simulink model " PV_PEM_indirect"  (R2026a)
settings: Solver=ode15s  StopTime=sim_t  MaxStep=1e-5
values from neighbouring files (symbols this model uses):
  Ra_stack = Ra   * N    (= 0.02301)    [ PV_PEM_indirect.m]    (also in PV_PEM_indirect.m = 0.02832)
  Rc_stack = Rc   * N    (= 0.0065)    [ PV_PEM_indirect.m]    (also in PV_PEM_indirect.m = 0.008)
  Rint_stack = Rint * N    (= 0.112749)    [ PV_PEM_indirect.m]    (also in PV_PEM_indirect.m = 0.138768)
  sample_output_time = 1e-2    (= 0.01)    [ PV_PEM_indirect.m]    (also in PV_PEM_indirect.m = Irr_stair_tsamp)
  Ts = Irr_stair_tsamp / N_sw_per_step    [PV_PEM_indirect.m]
  Tsc = 1e-5    (= 1e-05)    [ PV_PEM_indirect.m]    (also in PV_PEM_indirect.m = 5e-05)
libraries: fl_lib x16, nesl_utility x15, ee_lib x3, simulink x2, eeDcDcVoltageController x1, eePwmGenerator x1
settings Model: SimulationMode=accelerator  Creator=hanna  LastModifiedBy=Diamantis
settings SimscapeCC: SimscapeNominalValues="[{\"value\":\"1\",\"unit\":\"A\"},{\"value\":\"1\",\"unit\":\"bar\"},{\"value\":\"1\",\"unit\":\"cm^2\"},{\"value\":\"1\",\"unit\":\"cm^3/s\"},{\"value\":\"1\",\"unit\":\"kJ/kg\"},{\"value\":\"1\",\"unit\":\"kW\"},{\"value\":\"1\",\"unit\":\"l\"},{\"value\":\"1\",\"unit\":\"N\"},{\"value\":\"1\",\"unit\":\"N*m\"},{\"value\":\"1\",\"unit\":\"V\"}]"  SimscapeLogType=none  SimscapeLogDataHistory=5000.0

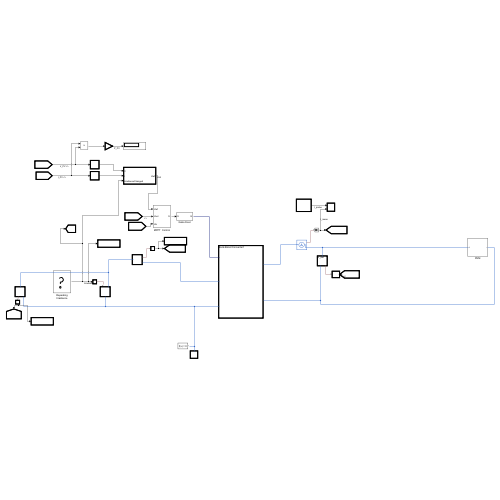
[thumbnail: Simulink's stored preview of the top-level diagram]
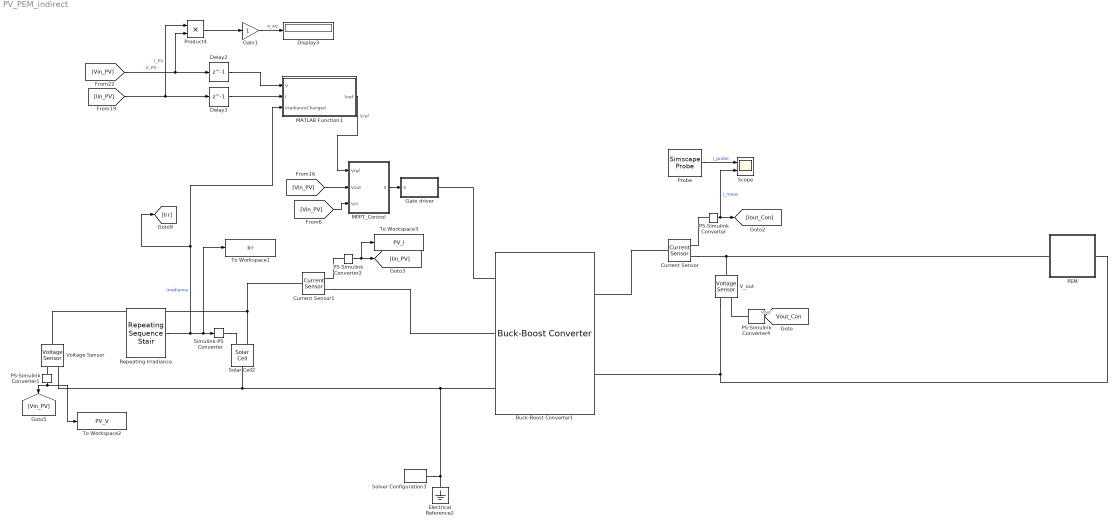
== system  PV_PEM_indirect ==
  Buck-Boost Converter1 : ee_lib/Semiconductors & Converters/Converters/Buck-Boost Converter  port_option=ee.enum.controlport.ps  device_type=4  Vf=0.8 V  Ron=0.001 Ohm  Rds=Ron Ohm  Goff=Conductance 1/Ohm  Vgt=1 V  Vgt_off=-1 V  Ih=1 A  Vth=Vth V  K=0  diode_param=2  diode_Vf=Vforward V  diode_Ron=1e-9 Ohm  diode_Goff=1e-6 1/Ohm  diode_C=50 nF  diode_iRM=5 A  diode_iF=300 A  diode_idot=-50 A/us  diode_trr_param=1  diode_trr_factor=3  diode_trr=0.5 us  diode_Qrr=1500 s*uA  Lf=L_conv H  Rl=0 Ohm  Cf=C_conv F  Rf=0 Ohm  snubber_type=1  Cs=1e-7 F  Rs=0.1 Ohm  iL_specify=off  iL_priority=High  iL=0 A  iL_nominal_specify=off  iL_nominal_value=1  iL_nominal_unit=A  vc_specify=off  vc_priority=High  vc=0 V  vc_nominal_specify=off  vc_nominal_value=1  vc_nominal_unit=V
  Current Sensor : fl_lib/Electrical/Electrical Sensors/Current Sensor
  Current Sensor1 : fl_lib/Electrical/Electrical Sensors/Current Sensor
  Delay2 : Delay  DelayLength=1
  Delay3 : Delay  DelayLength=1
  Display3 : Display
  Electrical Reference2 : fl_lib/Electrical/Electrical Elements/Electrical Reference
  Gain1 : Gain
  Gate driver : Subsystem
  MATLAB Function1 : MATLAB Function  TreatAsAtomicUnit=on
  MPPT_Control : Subsystem
  PEM : Subsystem
  PS-Simulink Converter : nesl_utility/PS-Simulink Converter  PhysicalDomain=network_engine_domain  SubClassName=ps_output  LeftPortType=input  RightPortType=output  PseudoPeriodic=off  Frequencies=[]  VectorFormat=inherit  Unit=inherit  AffineConversion=off
  PS-Simulink Converter1 : nesl_utility/PS-Simulink Converter  PhysicalDomain=network_engine_domain  SubClassName=ps_output  LeftPortType=input  RightPortType=output  PseudoPeriodic=off  Frequencies=[]  VectorFormat=inherit  Unit=inherit  AffineConversion=off
  PS-Simulink Converter2 : nesl_utility/PS-Simulink Converter  PhysicalDomain=network_engine_domain  SubClassName=ps_output  LeftPortType=input  RightPortType=output  PseudoPeriodic=off  Frequencies=[]  VectorFormat=inherit  Unit=inherit  AffineConversion=off
  PS-Simulink Converter4 : nesl_utility/PS-Simulink Converter  PhysicalDomain=network_engine_domain  SubClassName=ps_output  LeftPortType=input  RightPortType=output  PseudoPeriodic=off  Frequencies=[]  VectorFormat=1-D array  Unit=V  AffineConversion=off
  Probe : SimscapeProbe  BoundBlock=1212  Variables="{\"I\":{\"Probing\":\"ON\"}}"
  Product4 : Product
  Repeating Irradiance : simulink/Sources/Repeating Sequence Stair  OutValues=Irr_stair_val  tsamp=Irr_stair_tsamp  OutMin=[]  OutMax=[]  OutDataTypeStr=double  OutputDataTypeScalingMode=double  OutDataType=fixdt(0,8)  ConRadixGroup=Best Precision: Vector-wise  OutScaling=2^-12
  Scope : Scope  NumInputPorts=2
  Simulink-PS Converter : nesl_utility/Simulink-PS Converter  PhysicalDomain=network_engine_domain  SubClassName=ps_input  LeftPortType=input  RightPortType=output  PseudoPeriodic=off  Frequencies=[]  NoiseDistribution=none  NoiseParameters=[]  Unit=1  AffineConversion=off  FilteringAndDerivatives=provide  SimscapeFilterOrder=1  InputFilterTimeConstant=0.001  UdotUserProvided=0
  Solar Cell2 : ee_lib/Sources/Solar Cell  PartSpecification="{\"CollectionId\":\"SimscapeElectrical\",\"CollectionVersion\":\"1.0.0\",\"DatasetId\":\"Amerisolar|AS_6M30_HC_320W|simscape.electrical.solarCell\",\"DisplayName\":\"Amerisolar:AS_6M30_HC_320W\"}"  prm=3  Isc=10.14 % Datasheet derived A  Voc=0.67 % Datasheet derived V  Is=3.24823447983853e-07 % Datasheet derived A  Is2=9.37081970792037e-10 % Datasheet derived A  Iph=10.140005507508 % Datasheet derived A  Ir0=1000 % Datasheet derived W/m^2  ec=1.51118472243322 % Datasheet derived  N2=2.60259908345858 % Datasheet derived  Rs=1.94548269975201e-05 % Datasheet derived Ohm  Rp=682.95993142779 % Datasheet derived Ohm  N_series=Ns_cell % Datasheet derived  N_parallel=Np_cell % Datasheet derived  TIPH1=0.000499942933005141 % Datasheet derived 1/K  EG=1.12 % Datasheet derived eV  TXIS1=4.23641510120988 % Datasheet derived  TXIS2=16.2689137700667 % Datasheet derived  TRS1=0.243341028305912 % Datasheet derived  TRP1=0 % Parameter not set  Tmeas=25 % Datasheet derived degC  TFIXED=25 % Datasheet derived degC  thermal_mass=100 % Parameter not set J/K  initial_temperature=25 degC
      settings: AttributesFormatString=Amerisolar:AS_6M30_HC_320W
  Solver Configuration3 : nesl_utility/Solver Configuration  PhysicalDomain=network_engine_domain  SubClassName=solver  LeftPortType=input  RightPortType=generic  Tones=[]  Harmonics=[]  SimulateNoise=off  Profile=off  UseLocalSampling=off  EnableSwitchedLinearOptims=on  FrequencyDomain=off  UseCCode=off  RelTol=0.001  AbsTol=1e-06  MinStep=1e-09  ToWorkspace=off  RevertToSquareIcSolve=off  NumHomotopyIterations=100  PhasorMode=off  PhasorModeNumHarmonics=1  ConsistencySolver=NEWTON_FTOL  CanonicalOrdering=UNORDERED  OptimizeIntermediates=UNOPTIMIZED  IndexReductionMethod=DerivativeReplacement  DoDC=off  ResidualTolerance=1e-3  ConsistencyTolSource=GLOBAL  ConsistencyAbsTol=0.001  ConsistencyRelTol=0.001  ConsistencyTolFactor=0.001  UseLocalSolver=off  LocalSolverChoice=NE_BACKWARD_EULER_ADVANCER  ResolveIndetEquations=on  FunctionEvalNumThread=1  LocalSolverSampleTime=1e-5  DoFixedCost=off  MaxNonlinIter=2  MaxModeIter=2  ComputeImpulses=off  ImpulseIterations=2  LinearAlgebra=Sparse  LinearAlgebraNumThread=0  EquationFormulation=NE_TIME_EF  DelaysMemoryBudget=1024  AutomaticFiltering=on  FilteringTimeConstant=10e-7  PartitionStorageMethod=AS_NEEDED  PartitionMemoryBudget=1024  PartitionMethod=ROBUST  MultibodyUseLocalSolver=off  MultibodyLocalSolverChoice=ODE1  MultibodyLocalSolverSampleTime=0.001
  To Workspace1 : ToWorkspace  VariableName=Irr  SaveFormat=Timeseries  SampleTime=sample_output_time
  To Workspace2 : ToWorkspace  VariableName=PV_V  SaveFormat=Timeseries  SampleTime=sample_output_time
  To Workspace3 : ToWorkspace  VariableName=PV_I  SaveFormat=Timeseries  SampleTime=sample_output_time
  V_out : fl_lib/Electrical/Electrical Sensors/Voltage Sensor
  Voltage Sensor : fl_lib/Electrical/Electrical Sensors/Voltage Sensor
  tag scope: Vout_Con=global
  wires:
  PS-Simulink Converter1/1 -> [Vin_PV], To Workspace2/1
  Repeating Irradiance/1 -> [Irr], MATLAB Function1/3(irradianceChanged), Simulink-PS Converter/1, To Workspace1/1  "Irradiance"
  PS-Simulink Converter/1 -> Scope/2, [Iout_Con]  "I_meas"
  PS-Simulink Converter4/1 -> [Vout_Con]  "Vout"
  PS-Simulink Converter2/1 -> To Workspace3/1, [Iin_PV]
  Delay2/1 -> MATLAB Function1/1(V)
  Product4/1 -> Gain1/1
  [Vin_PV] -> Delay2/1, Product4/2  "V_PV"
  [Iin_PV] -> Product4/1, Delay3/1  "I_PV"
  Gain1/1 -> Display3/1  "P_PV"
  Delay3/1 -> MATLAB Function1/2(I)
  MPPT_Control/1(S) -> Gate driver/1(S)
  MATLAB Function1/1(Vref) -> MPPT_Control/1(Vref)  "Vref"
  [Vin_PV] -> MPPT_Control/2(Vout)
  [Vin_PV] -> MPPT_Control/3(Vin)
  Probe/1 -> Scope/1  "I_probe"
  connections:
  Electrical Reference2/LConn1 -- Solver Configuration3/RConn1 -- Voltage Sensor/RConn2 -- Solar Cell2/RConn1 -- Buck-Boost Converter1/LConn3
  Voltage Sensor/LConn1 -- Solar Cell2/LConn2 -- Current Sensor1/LConn1
  Buck-Boost Converter1/LConn1 -- Gate driver/RConn1
  PS-Simulink Converter1/LConn1 -- Voltage Sensor/RConn1
  Simulink-PS Converter/RConn1 -- Solar Cell2/LConn1
  PEM/LConn1 -- Current Sensor/RConn2 -- V_out/LConn1
  V_out/RConn2 -- PEM/RConn1 -- Buck-Boost Converter1/RConn2
  PS-Simulink Converter/LConn1 -- Current Sensor/RConn1
  Current Sensor/LConn1 -- Buck-Boost Converter1/RConn1
  PS-Simulink Converter4/LConn1 -- V_out/RConn1
  Current Sensor1/RConn2 -- Buck-Boost Converter1/LConn2
  PS-Simulink Converter2/LConn1 -- Current Sensor1/RConn1

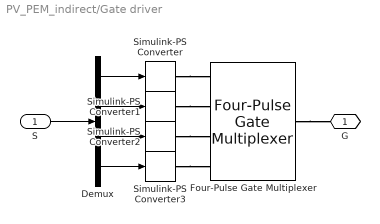
== system  PV_PEM_indirect/Gate driver ==
  S : Inport
  Demux : Demux
  Four-Pulse Gate Multiplexer : ee_lib/Semiconductors & Converters/Converters/Four-Pulse Gate Multiplexer  port_option=ee.enum.controlport.ps
  Simulink-PS Converter{,1..3} (4 alike) : nesl_utility/Simulink-PS Converter  PhysicalDomain=network_engine_domain  SubClassName=ps_input  LeftPortType=input  RightPortType=output  PseudoPeriodic=off  Frequencies=[]  NoiseDistribution=none  NoiseParameters=[]  Unit=1  AffineConversion=off  FilteringAndDerivatives=provide  SimscapeFilterOrder=1  InputFilterTimeConstant=0.001  UdotUserProvided=0
  G : PMIOPort  Side=Right
  wires:
  S/1 -> Demux/1
  Demux/1 -> Simulink-PS Converter/1
  Demux/2 -> Simulink-PS Converter1/1
  Demux/3 -> Simulink-PS Converter2/1
  Demux/4 -> Simulink-PS Converter3/1
  connections:
  Four-Pulse Gate Multiplexer/RConn1 -- G/RConn1
  Simulink-PS Converter/RConn1 -- Four-Pulse Gate Multiplexer/LConn1
  Simulink-PS Converter3/RConn1 -- Four-Pulse Gate Multiplexer/LConn4
  Simulink-PS Converter2/RConn1 -- Four-Pulse Gate Multiplexer/LConn3
  Simulink-PS Converter1/RConn1 -- Four-Pulse Gate Multiplexer/LConn2

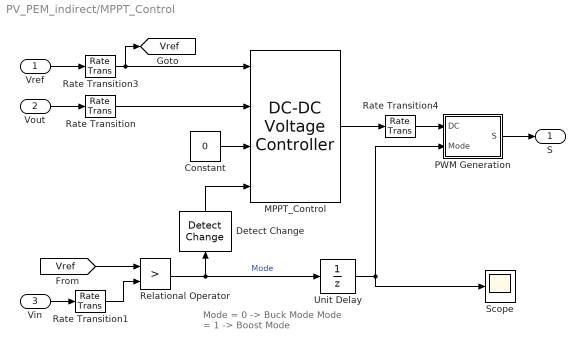
== system  PV_PEM_indirect/MPPT_Control ==
  note: Mode = 0 -> Buck Mode
      | Mode = 1 -> Boost Mode
  Vref : Inport
  Vout : Inport  Port=2
  Vin : Inport  Port=3
  Constant : Constant  Value=0
  Detect Change : simulink/Logic and Bit Operations/Detect Change  vinit=0  OutDataTypeStr=boolean
  MPPT_Control : eeDcDcVoltageController/DC-DC Voltage Controller  Kp=0.01  Ki=10.0  Kaw=1  upperLimit=0.60  lowerLimit=0  Ts=Ts  Tf=0.001  ActVdcFilter=off
  PWM Generation : Subsystem
  Rate Transition : RateTransition  OutPortSampleTime=Ts
  Rate Transition1 : RateTransition  OutPortSampleTime=Ts
  Rate Transition3 : RateTransition  OutPortSampleTime=Ts
  Rate Transition4 : RateTransition  OutPortSampleTime=Tsc
  Relational Operator : RelationalOperator  Operator=>  OutDataTypeStr=boolean  RndMeth=Simplest  InputSameDT=off
  Scope : Scope
      settings: ActiveDisplayYMinimum=-0.12499999999999997  ActiveDisplayYMaximum=1.125
  Unit Delay : UnitDelay  SampleTime=Tsc
  S : Outport  VectorParamsAs1DForOutWhenUnconnected=off
  tag scope: Vref=global
  wires:
  Vref/1 -> Rate Transition3/1
  Rate Transition3/1 -> MPPT_Control/1, [Vref]
  Vout/1 -> Rate Transition/1
  Rate Transition4/1 -> PWM Generation/1(DC)
  Rate Transition/1 -> MPPT_Control/2
  PWM Generation/1(S) -> S/1
  Vin/1 -> Rate Transition1/1
  MPPT_Control/1 -> Rate Transition4/1
  [Vref] -> Relational Operator/1
  Relational Operator/1 -> Unit Delay/1, Detect Change/1  "Mode"
  Rate Transition1/1 -> Relational Operator/2
  Detect Change/1 -> MPPT_Control/4
  Constant/1 -> MPPT_Control/3
  Unit Delay/1 -> PWM Generation/2(Mode), Scope/1

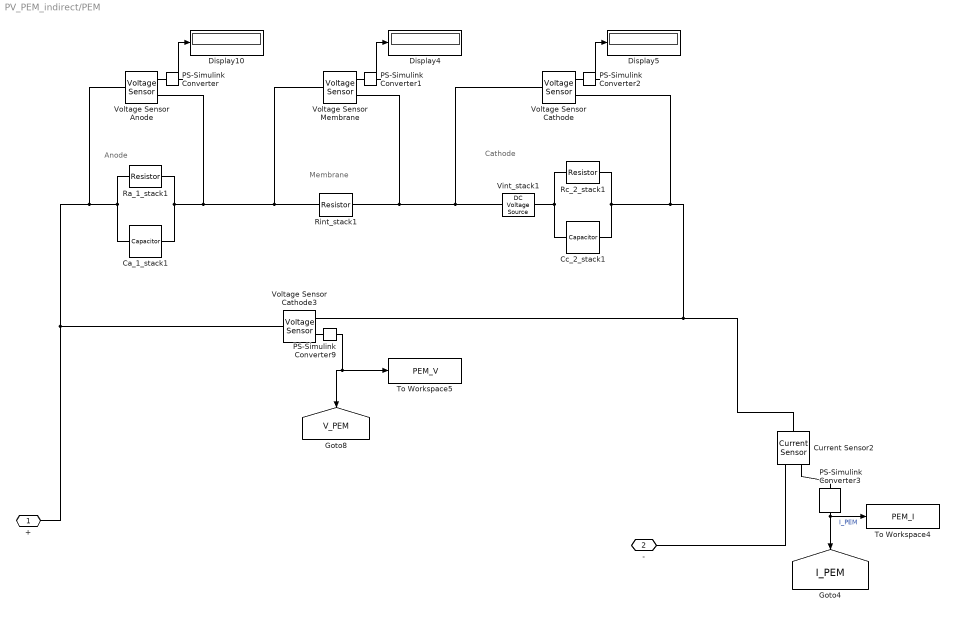
== system  PV_PEM_indirect/PEM ==
  note: Membrane
  note: Cathode
  note: Anode
  Ca_1_stack1 : fl_lib/Electrical/Electrical Elements/Capacitor  c=Ca_stack F  r=1e-6 Ohm  g=0 1/Ohm  i_specify=off  i_priority=None  i=0 A  i_nominal_specify=off  i_nominal_value=1  i_nominal_unit=A  v_specify=off  v_priority=None  v=0 V  v_nominal_specify=off  v_nominal_value=1  v_nominal_unit=V  vc_specify=off  vc_priority=High  vc=0 V  vc_nominal_specify=off  vc_nominal_value=1  vc_nominal_unit=V
  Cc_2_stack1 : fl_lib/Electrical/Electrical Elements/Capacitor  c=Cc_stack F  r=1e-6 Ohm  g=0 1/Ohm  i_specify=off  i_priority=None  i=0 A  i_nominal_specify=off  i_nominal_value=1  i_nominal_unit=A  v_specify=off  v_priority=None  v=0 V  v_nominal_specify=off  v_nominal_value=1  v_nominal_unit=V  vc_specify=off  vc_priority=High  vc=0 V  vc_nominal_specify=off  vc_nominal_value=1  vc_nominal_unit=V
  Current Sensor2 : fl_lib/Electrical/Electrical Sensors/Current Sensor
  Display10 : Display
  Display4 : Display
  Display5 : Display
  PS-Simulink Converter{,1..2,9} (4 alike) : nesl_utility/PS-Simulink Converter  PhysicalDomain=network_engine_domain  SubClassName=ps_output  LeftPortType=input  RightPortType=output  PseudoPeriodic=off  Frequencies=[]  VectorFormat=inherit  Unit=inherit  AffineConversion=off
  PS-Simulink Converter3 : nesl_utility/PS-Simulink Converter  PhysicalDomain=network_engine_domain  SubClassName=ps_output  LeftPortType=input  RightPortType=output  PseudoPeriodic=off  Frequencies=[]  VectorFormat=1-D array  Unit=mA  AffineConversion=off
  Ra_1_stack1 : fl_lib/Electrical/Electrical Elements/Resistor  R=Ra_stack Ohm  i_specify=off  i_priority=None  i=0 A  i_nominal_specify=off  i_nominal_value=1  i_nominal_unit=A  v_specify=off  v_priority=None  v=0 V  v_nominal_specify=off  v_nominal_value=1  v_nominal_unit=V
  Rc_2_stack1 : fl_lib/Electrical/Electrical Elements/Resistor  R=Rc_stack Ohm  i_specify=off  i_priority=None  i=0 A  i_nominal_specify=off  i_nominal_value=1  i_nominal_unit=A  v_specify=off  v_priority=None  v=0 V  v_nominal_specify=off  v_nominal_value=1  v_nominal_unit=V
  Rint_stack1 : fl_lib/Electrical/Electrical Elements/Resistor  R=Rint_stack Ohm  i_specify=off  i_priority=None  i=0 A  i_nominal_specify=off  i_nominal_value=1  i_nominal_unit=A  v_specify=off  v_priority=None  v=0 V  v_nominal_specify=off  v_nominal_value=1  v_nominal_unit=V
  To Workspace4 : ToWorkspace  VariableName=PEM_I  SaveFormat=Timeseries  SampleTime=sample_output_time
  To Workspace5 : ToWorkspace  VariableName=PEM_V  SaveFormat=Timeseries  SampleTime=sample_output_time
  Vint_stack1 : fl_lib/Electrical/Electrical Sources/DC Voltage Source  v0=Vint_stack V
  Voltage Sensor Anode : fl_lib/Electrical/Electrical Sensors/Voltage Sensor
  Voltage Sensor Cathode : fl_lib/Electrical/Electrical Sensors/Voltage Sensor
  Voltage Sensor Cathode3 : fl_lib/Electrical/Electrical Sensors/Voltage Sensor
  Voltage Sensor Membrane : fl_lib/Electrical/Electrical Sensors/Voltage Sensor
  + : PMIOPort  Side=Left
  - : PMIOPort  Port=2  Side=Right
  tag scope: I_PEM=global, V_PEM=global
  wires:
  PS-Simulink Converter/1 -> Display10/1
  PS-Simulink Converter1/1 -> Display4/1
  PS-Simulink Converter2/1 -> Display5/1
  PS-Simulink Converter3/1 -> [I_PEM], To Workspace4/1  "I_PEM"
  PS-Simulink Converter9/1 -> [V_PEM], To Workspace5/1
  connections:
  Rint_stack1/LConn1 -- Voltage Sensor Membrane/LConn1 -- Ra_1_stack1/RConn1 -- Ca_1_stack1/RConn1 -- Voltage Sensor Anode/RConn2
  Voltage Sensor Cathode3/RConn2 -- Current Sensor2/LConn1 -- Voltage Sensor Cathode/RConn2 -- Rc_2_stack1/RConn1 -- Cc_2_stack1/RConn1
  Voltage Sensor Cathode/RConn1 -- PS-Simulink Converter2/LConn1
  Vint_stack1/RConn1 -- Rc_2_stack1/LConn1 -- Cc_2_stack1/LConn1
  Ca_1_stack1/LConn1 -- Ra_1_stack1/LConn1 -- +/RConn1 -- Voltage Sensor Cathode3/LConn1 -- Voltage Sensor Anode/LConn1
  Voltage Sensor Cathode/LConn1 -- Rint_stack1/RConn1 -- Voltage Sensor Membrane/RConn2 -- Vint_stack1/LConn1
  Voltage Sensor Cathode3/RConn1 -- PS-Simulink Converter9/LConn1
  Voltage Sensor Anode/RConn1 -- PS-Simulink Converter/LConn1
  Voltage Sensor Membrane/RConn1 -- PS-Simulink Converter1/LConn1
  Current Sensor2/RConn1 -- PS-Simulink Converter3/LConn1
  Current Sensor2/RConn2 -- -/RConn1

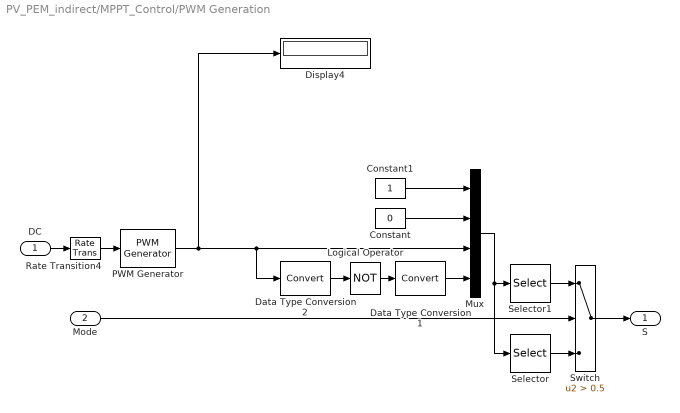
== system  PV_PEM_indirect/MPPT_Control/PWM Generation ==
  DC : Inport
  Mode : Inport  Port=2
  Constant : Constant  Value=0
  Constant1 : Constant
  Data Type Conversion1 : DataTypeConversion  SaturateOnIntegerOverflow=off  RndMeth=Floor
  Data Type Conversion2 : DataTypeConversion  SaturateOnIntegerOverflow=off  RndMeth=Floor
  Display4 : Display
  Logical Operator : Logic  Operator=NOT  AllPortsSameDT=off  OutDataTypeStr=boolean
  Mux : Mux
  PWM Generator : eePwmGenerator/PWM Generator  CarrCount=Up  Tper=Ts  Tdelay=0  Ts=Tsc
  Rate Transition4 : RateTransition  OutPortSampleTime=Tsc
  Selector : Selector  InputPortWidth=4  IndexOptions=Index vector (dialog)  Indices=[3 4 2 1]  OutputSizes=1
  Selector1 : Selector  InputPortWidth=4  IndexOptions=Index vector (dialog)  Indices=[1:4]  OutputSizes=1
  Switch : Switch  Criteria=u2 > Threshold  Threshold=0.5  SaturateOnIntegerOverflow=off  InputSameDT=off
  S : Outport  VectorParamsAs1DForOutWhenUnconnected=off
  wires:
  Rate Transition4/1 -> PWM Generator/1
  Logical Operator/1 -> Data Type Conversion1/1
  DC/1 -> Rate Transition4/1
  Data Type Conversion2/1 -> Logical Operator/1
  Mode/1 -> Switch/2
  Selector1/1 -> Switch/1
  Selector/1 -> Switch/3
  Mux/1 -> Selector/1, Selector1/1
  Switch/1 -> S/1
  Data Type Conversion1/1 -> Mux/4
  Constant/1 -> Mux/2
  Constant1/1 -> Mux/1
  PWM Generator/1 -> Display4/1, Mux/3, Data Type Conversion2/1

== matlab function  PV_PEM_indirect/MATLAB Function1 ==
  data: V input; Vref output; I input; irradianceChanged input
function Vref = RefGen(V, I, irradianceChanged)
    % Define constants
    Vrefmax = 1000;
    Vrefmini = 0;
    Vrefinit = 500;
    
    baseDeltaVref = 1; % Base step size
    
    % Persistent variables to store previous values
    persistent Vold Pold Vrefold deltaVref;
    
    % Initialize persistent variables if they are empty or irradiance changed
    if isempty(Vold) || irradianceChanged
        Vold = 0;
        Pold = 0;
        Vrefold = Vrefinit;
        deltaVref = baseDeltaVref; % Reset to base step size
    end
    
    % Calculate current power
    P = V * I;
    dV = V - Vold;
    dP = P - Pold;
    
    % Adjust Vref based on dP and dV
    if dP ~= 0
        if dP < 0
            if dV < 0
                Vref = Vrefold + deltaVref;
            else
                Vref = Vrefold - deltaVref;
            end
        else
            if dV < 0
                Vref = Vrefold - deltaVref;
            else
                Vref = Vrefold + deltaVref;
            end
        end
        
        % Adaptive step size: Increase step size if power change is large
        deltaVref = baseDeltaVref * (1 + abs(dP) / P);
    else
        Vref = Vrefold;
        % Reduce step size if no significant power change
        deltaVref = max(baseDeltaVref, deltaVref * 0.9);
    end
    
    % Constrain Vref within bounds
    if Vref >= Vrefmax
        Vref = Vrefmax;
    elseif Vref <= Vrefmini
        Vref = Vrefmini;
    end
    
    % Update persistent variables for next iteration
    Vrefold = Vref;
    Vold = V;
    Pold = P;
end
